simulink model "hw_v"  (R2022b)
settings: Solver=VariableStepAuto  StartTime=0.0  StopTime=10.0  RelTol=1e-3
settings Model: Creator=Wasif  LastModifiedBy=Wasif

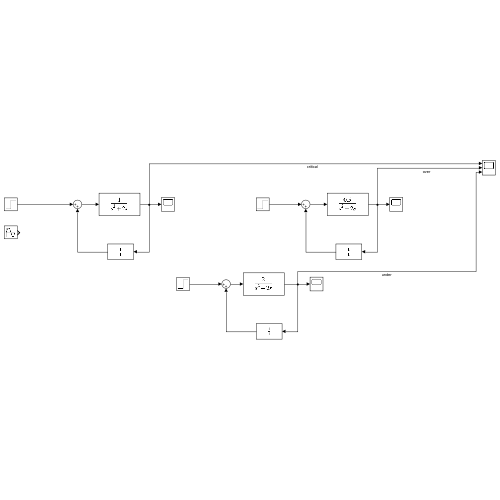
[thumbnail: Simulink's stored preview of the top-level diagram]
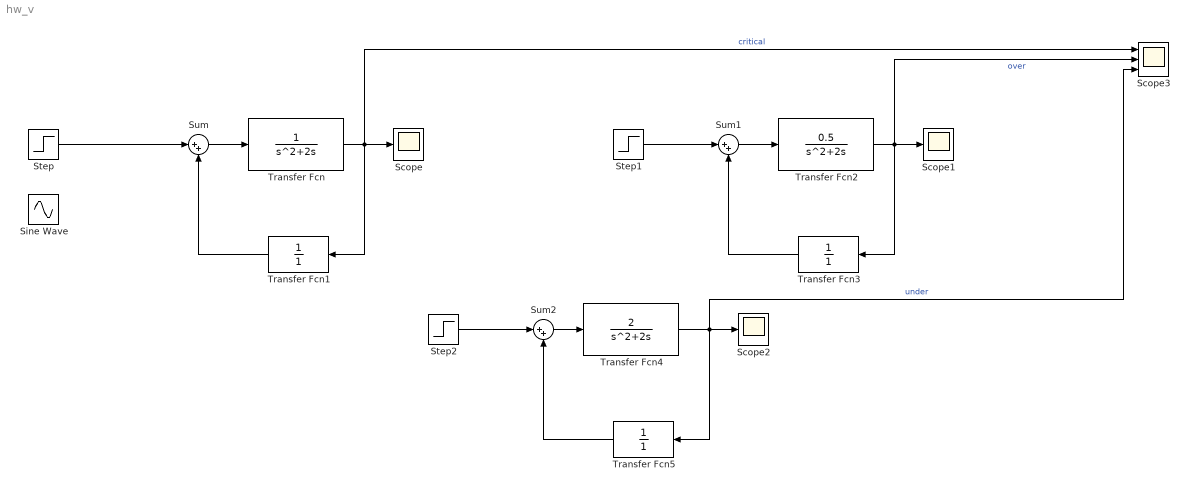
== system hw_v ==
  Scope : Scope
  Scope1 : Scope
  Scope2 : Scope
  Scope3 : Scope  NumInputPorts=3
  Sine Wave : Sin  SampleTime=0
  Step : Step  SampleTime=0
  Step1 : Step  SampleTime=0
  Step2 : Step  SampleTime=0
  Sum : Sum  Inputs=|++
  Sum1 : Sum  Inputs=|++
  Sum2 : Sum  Inputs=|++
  Transfer Fcn : TransferFcn  Denominator=[1 2 0]
  Transfer Fcn1 : TransferFcn  Denominator=[ 1]
  Transfer Fcn2 : TransferFcn  Numerator=[0.5]  Denominator=[1 2 0]
  Transfer Fcn3 : TransferFcn  Denominator=[ 1]
  Transfer Fcn4 : TransferFcn  Numerator=[2]  Denominator=[1 2 0]
  Transfer Fcn5 : TransferFcn  Denominator=[ 1]
  wires:
  Transfer Fcn/1 -> Scope3/1, Transfer Fcn1/1, Scope/1  "critical"
  Transfer Fcn1/1 -> Sum/2
  Sum/1 -> Transfer Fcn/1
  Sum1/1 -> Transfer Fcn2/1
  Step1/1 -> Sum1/1
  Transfer Fcn2/1 -> Scope3/2, Transfer Fcn3/1, Scope1/1  "over"
  Transfer Fcn3/1 -> Sum1/2
  Sum2/1 -> Transfer Fcn4/1
  Step2/1 -> Sum2/1
  Transfer Fcn4/1 -> Scope3/3, Transfer Fcn5/1, Scope2/1  "under"
  Transfer Fcn5/1 -> Sum2/2
  Step/1 -> Sum/1
